simulink model "PID_Controller"  (R2020b)
settings: Solver=VariableStepAuto  StartTime=0.0  StopTime=10.0  RelTol=1e-3
values from neighbouring files (symbols this model uses):
  Kd = 10.0    [Dict_Assignment_3.sldd]
  Ki = 70.0    [Dict_Assignment_3.sldd]
  Kp = 1500.0    [Dict_Assignment_3.sldd]
settings Model: DataDictionary=Dict_Assignment_3.sldd  Creator=Shantam Garg  LastModifiedBy=Shantam Garg
settings DataIOCC: SaveOutput=off  SaveTime=off

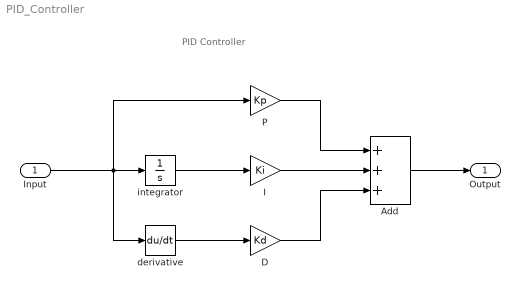
== system PID_Controller ==
  note: PID Controller
  Input : Inport  OutDataTypeStr=double  PortDimensions=1  SampleTime=0
  Add : Sum  Inputs=+++
  D : Gain  Gain=Kd
  I : Gain  Gain=Ki
  P : Gain  Gain=Kp
  derivative : Derivative
  integrator : Integrator
  Output : Outport  OutDataTypeStr=double  PortDimensions=1  SampleTime=0
  wires:
  Add/1 -> Output/1
  Input/1 -> integrator/1, P/1, derivative/1
  P/1 -> Add/1
  D/1 -> Add/3
  derivative/1 -> D/1
  integrator/1 -> I/1
  I/1 -> Add/2
